simulink model "motor_driver"  (R2022a)
settings: Solver=VariableStepAuto  StartTime=0.0  StopTime=1  MaxStep=1e-6  RelTol=1e-6
libraries: simulink x1
settings Model: Creator=User  LastModifiedBy=User

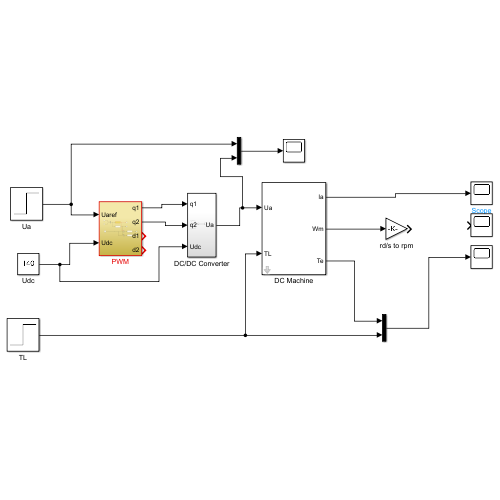
[thumbnail: Simulink's stored preview of the top-level diagram]
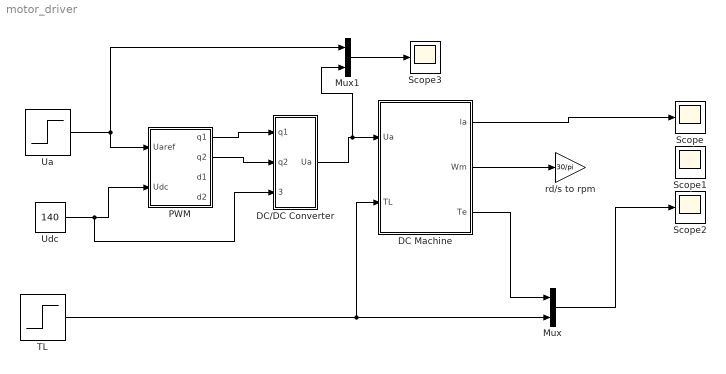
== system motor_driver ==
  DC Machine : Subsystem  mask{Ra=0.5, La=2.5e-3, J=1e-3, fr=5e-2, Ke=0.35, Kc=0.35}
      mask prompts: Ra "Ra(Ohm)"; La "La(H)"; J "J(N.m.s^-1)"; fr "fr(N.m.s)"; Ke "Ke(V.s)"; Kc "Kc(N.m.A^-1)"
  DC/DC Converter : Subsystem
  Mux : Mux  Inputs=2
  Mux1 : Mux  Inputs=2
  PWM : Subsystem
  Scope{,1..3} (4 alike) : Scope
  TL : Step  Time=0.5  After=7  SampleTime=0
  Ua : Step  Time=0.1  After=120  SampleTime=0
  Udc : Constant  Value=140
  rd/s to rpm : Gain  Gain=30/pi
  wires:
  DC Machine/2(Wm) -> rd/s to rpm/1
  PWM/1(q1) -> DC/DC Converter/1(q1)
  PWM/2(q2) -> DC/DC Converter/2(q2)
  DC/DC Converter/1(Ua) -> Mux1/2, DC Machine/1(Ua)
  DC Machine/1(la) -> Scope/1
  DC Machine/3(Te) -> Mux/1
  TL/1 -> DC Machine/2(TL), Mux/2
  Udc/1 -> DC/DC Converter/3(Udc), PWM/2(Udc)
  Ua/1 -> Mux1/1, PWM/1(Uaref)
  Mux/1 -> Scope2/1
  Mux1/1 -> Scope3/1

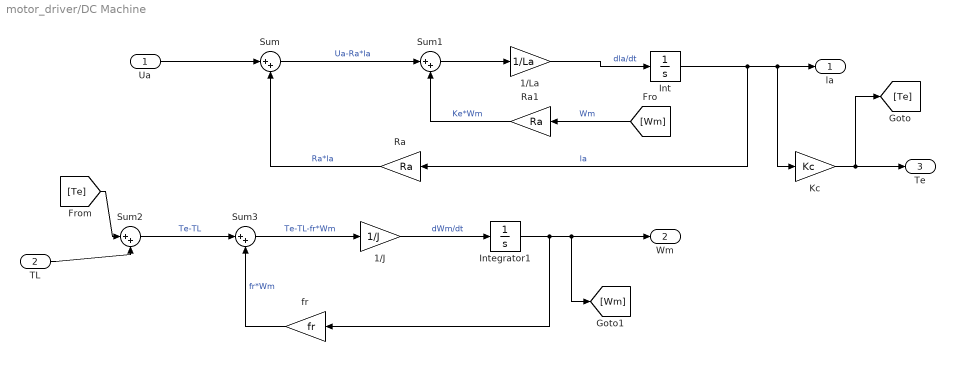
== system motor_driver/DC Machine ==
  Ua : Inport
  TL : Inport  Port=2
  1/J : Gain  Gain=1/J
  1/La : Gain  Gain=1/La
  Int : Integrator
  Integrator1 : Integrator
  Kc : Gain  Gain=Kc
  Ra : Gain  Gain=Ra
  Ra1 : Gain  Gain=Ra
  Sum{,1..3} (4 alike) : Sum  Inputs=|++
  fr : Gain  Gain=fr
  la : Outport
  Wm : Outport  Port=2
  Te : Outport  Port=3
  wires:
  [Wm] -> Ra1/1  "Wm"
  Sum1/1 -> 1/La/1
  Ra1/1 -> Sum1/2  "Ke*Wm"
  Kc/1 -> Te/1, [Te]
  1/J/1 -> Integrator1/1  "dWm/dt"
  Ra/1 -> Sum/2  "Ra*la"
  Integrator1/1 -> fr/1, Wm/1, [Wm]
  fr/1 -> Sum3/2  "fr*Wm"
  Sum3/1 -> 1/J/1  "Te-TL-fr*Wm"
  Sum2/1 -> Sum3/1  "Te-TL"
  Int/1 -> Ra/1, la/1, Kc/1  "la"
  TL/1 -> Sum2/2
  1/La/1 -> Int/1  "dla/dt"
  Ua/1 -> Sum/1
  Sum/1 -> Sum1/1  "Ua-Ra*la"
  [Te] -> Sum2/1

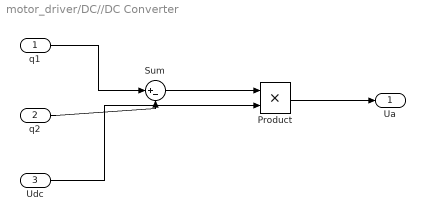
== system motor_driver/DC//DC Converter ==
  q1 : Inport
  q2 : Inport  Port=2
  Udc : Inport  Port=3
  Product : Product
  Sum : Sum  Inputs=|+-
  Ua : Outport
  wires:
  q1/1 -> Sum/1
  q2/1 -> Sum/2
  Udc/1 -> Product/2
  Sum/1 -> Product/1
  Product/1 -> Ua/1

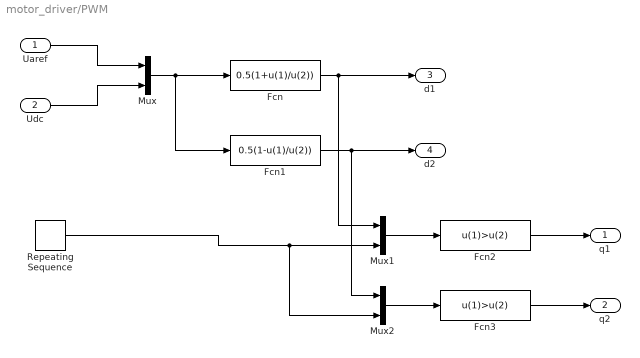
== system motor_driver/PWM ==
  Uaref : Inport
  Udc : Inport  Port=2
  Fcn : MATLABFcn  MATLABFcn=0.5(1+u(1)/u(2))
  Fcn1 : MATLABFcn  MATLABFcn=0.5(1-u(1)/u(2))
  Fcn2 : MATLABFcn  MATLABFcn=u(1)>u(2)
  Fcn3 : MATLABFcn  MATLABFcn=u(1)>u(2)
  Mux : Mux  Inputs=2
  Mux1 : Mux  Inputs=2
  Mux2 : Mux  Inputs=2
  Repeating Sequence : simulink/Sources/Repeating Sequence  rep_seq_t=[0 100e-6 200e-6]  rep_seq_y=[1 0 1]
  q1 : Outport
  q2 : Outport  Port=2
  d1 : Outport  Port=3
  d2 : Outport  Port=4
  wires:
  Uaref/1 -> Mux/1
  Udc/1 -> Mux/2
  Mux/1 -> Fcn1/1, Fcn/1
  Fcn1/1 -> Mux2/1, d2/1
  Fcn/1 -> Mux1/1, d1/1
  Repeating Sequence/1 -> Mux2/2, Mux1/2
  Mux1/1 -> Fcn2/1
  Mux2/1 -> Fcn3/1
  Fcn2/1 -> q1/1
  Fcn3/1 -> q2/1
